simulink model "SIMULINK"  (R2025b)
settings: Solver=ode45  StartTime=0.0  StopTime=0.005  MaxStep=1e-6  RelTol=1e-6
InitFcn:
  | L = 2e-3;
  | R = 10;
  | C = 10e-6;
  | Uin = 32;
  | f_pwn = 1003;
  | T = 1/f_pwn;
  | D = 0.40;
settings Model: Creator=andre  LastModifiedBy=andre

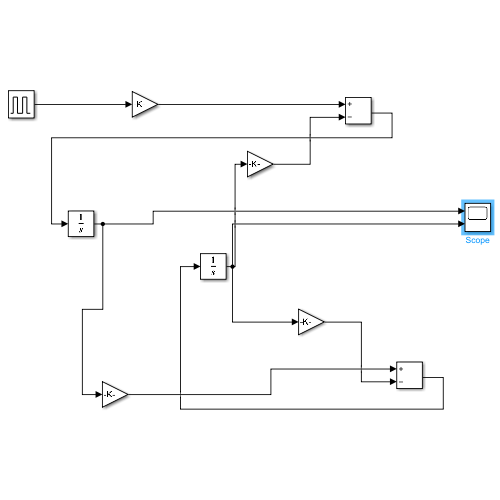
[thumbnail: Simulink's stored preview of the top-level diagram]
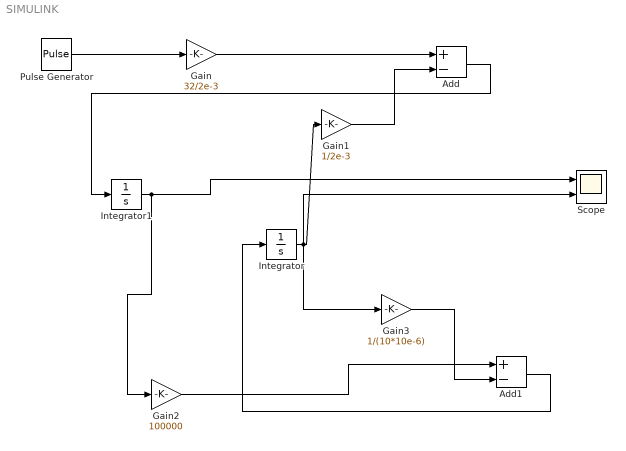
== system SIMULINK ==
  Add : Sum  Inputs=+-
  Add1 : Sum  Inputs=+-
  Gain : Gain  Gain=32/2e-3
  Gain1 : Gain  Gain=1/2e-3
  Gain2 : Gain  Gain=100000
  Gain3 : Gain  Gain=1/(10*10e-6)
  Integrator : Integrator
  Integrator1 : Integrator
  Pulse Generator : DiscretePulseGenerator  PulseType=Time based  Period=1/100e3  PulseWidth=40
  Scope : Scope  NumInputPorts=2
      settings: TimeUnits=Metric (based on Time Span)  ActiveDisplayYMinimum=-0.17312047082287454  ActiveDisplayYMaximum=1.5580842374058712
  wires:
  Pulse Generator/1 -> Gain/1
  Gain/1 -> Add/1
  Gain1/1 -> Add/2
  Add/1 -> Integrator1/1
  Integrator/1 -> Gain3/1, Scope/2, Gain1/1
  Integrator1/1 -> Gain2/1, Scope/1
  Add1/1 -> Integrator/1
  Gain3/1 -> Add1/2
  Gain2/1 -> Add1/1
